simulink model "VisionVehicleDetectorTestBench"  (R2024b)
settings: Solver=FixedStepAuto  StartTime=0.0  StopTime=scenario.StopTime  RelTol=1e-3
PostLoadFcn:
  | helperSLVisionVehicleDetectorSetup
values from neighbouring files (symbols this model uses):
  vehSim3D = repmat(         struct(             'Length', 0,             'RearOverhang', 0,             'InitialPos',[0 0 0],             'InitialRot',[0 0 0]),         numVehicles,1)    [helperSLVisionVehicleDetectorSetup.m]
undefined symbols (not defined in the file or in its folder): Sim3dSensor, Ts
libraries: drivingscenarioandsensors x8, sim3dautolib x6, sim3dcameralib x1, sim3dlib x1
CloseFcn:
  | helperSLVisionVehicleDetectorCleanUp
settings Model: SILPILSystemUnderTest=refmodels  Creator=The MathWorks, Inc.  LastModifiedBy=The MathWorks, Inc.
settings SolverCC: AlgebraicLoopSolver=TrustRegion  MaxZcPerStep=1
settings DataIOCC: SaveFormat=StructureWithTime  SaveOutput=off  DSMLogging=off  SaveTime=off
settings OptimizationCC: DefaultParameterBehavior=Inlined  EnhancedBackFolding=on  PassReuseOutputArgsAs=Individual arguments  ZeroExternalMemoryAtStartup=off  ZeroInternalMemoryAtStartup=off  InitFltsAndDblsToZero=on  OptimizeBlockOrder=speed  DifferentSizesBufferReuse=on  OptimizationCustomize=off  EfficientTunableParamExpr=on
settings DebuggingCC: ParameterTunabilityLossMsg=error  UnconnectedInputMsg=warning  UnconnectedOutputMsg=warning  UnconnectedLineMsg=warning  SubsystemReferenceDiagnosticForUnitTest=warning
settings HardwareCC: ProdLongLongMode=on  TargetLongLongMode=on
settings ModelReferenceCC: EnableRefExpFcnMdlSchedulingChecks=on
settings SFSimCC: SimTargetLang=C++
settings RTWCC: Description=Embedded Coder  SystemTargetFile=ert.tlc  TemplateMakefile=ert_default_tmf  CodeExecutionProfiling=on  CodeProfilingSaveOptions=AllData  TargetLang=C++  GPUComputeCapability=3.5  DLArmComputeVersion=19.05
settings CodeAppCC: ForceParamTrailComments=on  IgnoreCustomStorageClasses=off  OperatorAnnotations=on  SimulinkDataObjDesc=on  SFDataObjDesc=on  InsertBlockDesc=on
settings ERTTargetCC: TargetLangStandard=C++03 (ISO)  GenerateSampleERTMain=on  CodeInterfacePackaging=C++ class  SupportVariableSizeSignals=on  RootIOFormat=Structure reference  ERTCustomFileTemplate=example_file_process.tlc  DynamicArrayContainerType=coder::array
settings ConfigComp: CovScope=ReferencedModels  CovIncludeTopModel=off  CovExternalEMLEnable=off  CovSFcnEnable=off

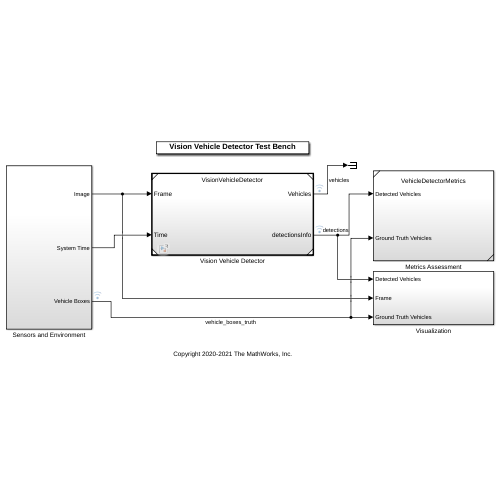
[thumbnail: Simulink's stored preview of the top-level diagram]
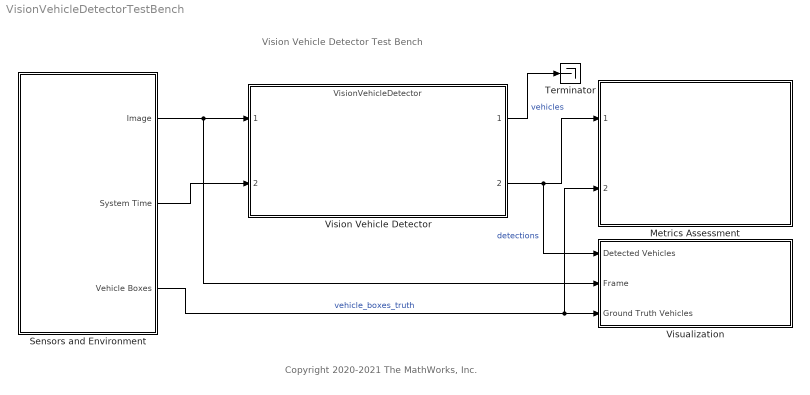
== system VisionVehicleDetectorTestBench ==
  note: Copyright 2020-2021 The MathWorks, Inc.
  note: Vision Vehicle Detector Test Bench
  Metrics Assessment : Subsystem  ReferencedSubsystem=VehicleDetectorMetrics
  Sensors and Environment : Subsystem
  Terminator : Terminator
  Vision Vehicle Detector : ModelReference  ModelNameDialog=VisionVehicleDetector.slx  SimulationMode=Normal  CodeInterface=Top model  ModelReferenceVersion=9.0
  Visualization : Subsystem
  wires:
  Sensors and Environment/3(Vehicle Boxes) -> Visualization/3(Ground Truth Vehicles), Metrics Assessment/2  "vehicle_boxes_truth"
  Sensors and Environment/1(Image) -> Vision Vehicle Detector/1, Visualization/2(Frame)
  Sensors and Environment/2(System Time) -> Vision Vehicle Detector/2
  Vision Vehicle Detector/1 -> Terminator/1  "vehicles"
  Vision Vehicle Detector/2 -> Metrics Assessment/1, Visualization/1(Detected Vehicles)  "detections"

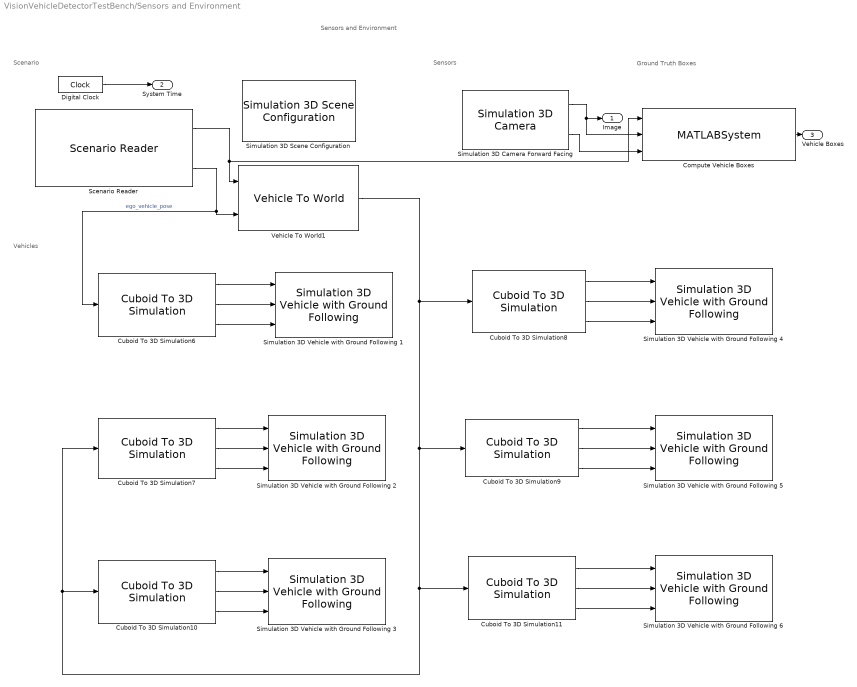
== system VisionVehicleDetectorTestBench/Sensors and Environment ==
  note: Sensors and Environment
  note: Ground Truth Boxes
  note: Sensors
  note: Vehicles
  note: Scenario
  Compute Vehicle Boxes : MATLABSystem  System=HelperComputeGroundTruthBoxes  VehicleDimensions=dimensions  Camera=camera  SimulateUsing=Interpreted execution
      mask Type: HelperComputeGroundTruthBoxes
      mask Display:
      | disp('HelperComputeGroundTruthBoxes');
      | port_label('input',1,'actorPositions');
      | port_label('input',2,'frame');
      | port_label('input',3,'labelledFrame');
      | port_label('output',1,'BBoxes');
  Cuboid To 3D Simulation10 : drivingscenarioandsensors/Cuboid To 3D Simulation  SpecifyActorID=on  ActorIDToConvert=3  SimulateUsing=Interpreted execution
  Cuboid To 3D Simulation11 : drivingscenarioandsensors/Cuboid To 3D Simulation  SpecifyActorID=on  ActorIDToConvert=6  SimulateUsing=Interpreted execution
  Cuboid To 3D Simulation6 : drivingscenarioandsensors/Cuboid To 3D Simulation  SpecifyActorID=off  ActorIDToConvert=1  SimulateUsing=Interpreted execution
  Cuboid To 3D Simulation7 : drivingscenarioandsensors/Cuboid To 3D Simulation  SpecifyActorID=on  ActorIDToConvert=2  SimulateUsing=Interpreted execution
  Cuboid To 3D Simulation8 : drivingscenarioandsensors/Cuboid To 3D Simulation  SpecifyActorID=on  ActorIDToConvert=4  SimulateUsing=Interpreted execution
  Cuboid To 3D Simulation9 : drivingscenarioandsensors/Cuboid To 3D Simulation  SpecifyActorID=on  ActorIDToConvert=5  SimulateUsing=Interpreted execution
  Digital Clock : DigitalClock  SampleTime=0.1
  Scenario Reader : drivingscenarioandsensors/Scenario Reader  ScenarioSource=From workspace  ScenarioFileName=dblLaneChangeDrivingScenario.mat  ScenarioVariableName=scenario  OutputCoordinateSystem=Vehicle coordinates  EgoVehicleSource=Scenario  EgoVehicleActorID=1  OrientVehiclesOnRoad=off  OutputEgoVehiclePose=on  OutputEgoVehicleState=off  SampleTime=0.1  LaneBoundaryOutput=None  LaneBoundaryDistance=0:0.5:70  LaneBoundaryLocation=Center of lane markings  BusNameSource=Auto  BusName=BusActors  BusNumActorsSource=Scenario  BusNumActors=100  BusName2Source=Auto  BusName2=BusLaneBoundaries  BusNumLaneBoundariesSource=Scenario  BusNumLaneBoundaries=10  BusName3Source=Auto  BusName3=BusEgoActor  BusName4Source=Auto  BusName4=BusEgoState  ShowCoordinateLabels=on  SimulateUsing=Interpreted execution
  Simulation 3D Camera Forward Facing : sim3dcameralib/Simulation 3D Camera  Priority=1  sensorTag=Sim3dSensor�  sensorId=1  sensorName=Sim3dSensor�  vehTagList={'Scene Origin';'SimulinkVehicle1';'SimulinkVehicle2';'SimulinkVehicle3';'SimulinkVehicle4';'SimulinkVehicle5';'SimulinkVehicle6'}  vehTag=SimulinkVehicle1  mountLoc=Origin  offsetFlag=on  tmountOffset=camera.PositionSim3d  extTmount=off  rmountOffset=camera.Rotation  extRmount=off  FocalLength=camera.FocalLength  OpticalCenter=camera.PrincipalPoint  ImageSize=camera.ImageSize  RadialDistortion=[0, 0]  TangentialDistortion=[0, 0]  SensorSkew=0  DepthOutportEnabled=off  SemanticOutportEnabled=on  TransformOutportEnabled=off  SampleTime=-1  mountPoint=[0.57 0 1.2]  mountOrientation=[0 0 0]  aMode=3  ID=1
      settings: LibrarySourceBlock=drivingsim3d/Simulation 3D Camera
      settings: AttributesFormatString=|
      | -------------------------------------
      | ImageSize = %<ImageSize>
      | OpticalCenter = %<OpticalCenter>
      | FocalLength = %<FocalLength>
      | RadialDistortion = %<RadialDistortion>
      | mountLoc = %<mountLoc>
      | tmountOffset = %<tmountOffset>
      | rmountOffset = %<rmountOffset>
  Simulation 3D Scene Configuration : sim3dlib/Simulation 3D Scene Configuration  Priority=0  ProjectFormat=Default Scenes  SceneDesc=Curved road  ProjectName=/mathworks/devel/bat/filer/batfs2566-0/Bdoc24b.2855429/build/runnable/matlab/toolbox/shared/sim3d_projects/automotive_project_linux/UE/LinuxNoEditor/VehicleSimulation.sh  ScenePath=/Game/Maps/HwStrght  EnableOpenDRIVE=off  vehTagList={'Scene Origin';'SimulinkVehicle1';'SimulinkVehicle2';'SimulinkVehicle3';'SimulinkVehicle4';'SimulinkVehicle5';'SimulinkVehicle6'}  vehTag=SimulinkVehicle1  FreeCameraInitialTranslation=[0, 0, 0]  FreeCameraDefaultInitialTranslation=[-6, 0, 2]  FreeCameraInitialRotation=[0, 0, 0]  FreeCameraDefaultInitialRotation=[0, -15, 0]  OpVisEn=off  Ts=0.1  EnableWindow=on  EnableRemoteAccess=off  EnableWeather=off  SunAzimuth=90  SunAltitude=40.0  EnableGeospatialSun=off  Latitude=0  Longitude=0  Date=2023-01-01  Time=10:30:00  GeoTimeZone=-5.0  SunDaylightSaving=off  wind=1  clouds=10  EnableVolumetricClouds=off  CloudCoverage=0  CloudAltitude=6  fog=0  rain=0  RaindropsEffect=off  SnowDensity=0  EnableGeospatial=off  UseTrueOrigin=off  OriginHeight=200  OriginLatitude=40.744652  OriginLongitude=-73.988864  MapStyle=Aerial  AdditionalAssetIDs=[]  UseAdvancedSunSky=off  SolarTime=11  TimeZone=-5  Day=21  Month=9  Year=2022  UseDaylightSavingTime=on  DSTStartDay=10  DSTStartMonth=3  DSTEndDay=3  DSTEndMonth=11  DSTSwitchHour=2  sensorTag=MainCamera2  sensorId=2  sensorName=MainCamera2  mountLoc=Origin  offsetFlag=off  tmountOffset=[0, 0, 0]  rmountOffset=[0, 0, 0]  HorizontalResolution=1280  VerticalResolution=720  HorizontalFOV=60  mountPoint=[0 0 0]  mountOrientation=[0 0 0]  aMode=3  ID=2  GeoTrigger=Inactive
      settings: AttributesFormatString=SceneName = %<SceneDesc>  LibrarySourceBlock=drivingsim3d/Simulation 3D Scene Configuration
  Simulation 3D Vehicle with Ground Following 1 : sim3dautolib/Simulation 3D Vehicle with Ground Following  Priority=-1  PassVehMesh=Sedan  MeshPath=/MathWorksSimulation/Vehicles/Muscle/Meshes/SK_MuscleCar.SK_MuscleCar  TrackWidth=1.9  WheelBase=3  WheelRadius=0.35  VehColor=Blue  InitialPos=vehSim3D(1).InitialPos  InitialRot=vehSim3D(1).InitialRot  ActorName=SimulinkVehicle1  SampleTime=-1  ActorType=SimulinkVehicle  ID=1  aMode=3  ActorTag=SimulinkVehicle1  CoordinateScheme=ISO  VehLightsControl=off  HeadlightColor=[ 1, 1, 1 ]  HighBeamIntensity=100000  LowBeamIntensity=60000  HighBeamConeAngle=70  LowBeamConeAngle=70  LeftHeadlightOrientation=[ 0, 0 ]  RightHeadlightOrientation=[ 0, 0 ]  BrakelightIntensity=500  ReverselightIntensity=500  SignallightIntensity=500  SignallightPeriod=1  SignalPulseWidth=50  TransformOutportEnabled=off
      settings: LibrarySourceBlock=drivingsim3d/Simulation 3D Vehicle with Ground Following
      settings: AttributesFormatString=|
      | --------------------------------------
      | ActorName = %<ActorName>
      | PassVehMesh = %<PassVehMesh>
      | VehColor = %<VehColor>
  Simulation 3D Vehicle with Ground Following 2 : sim3dautolib/Simulation 3D Vehicle with Ground Following  Priority=-1  PassVehMesh=Sedan  MeshPath=/MathWorksSimulation/Vehicles/Muscle/Meshes/SK_MuscleCar.SK_MuscleCar  TrackWidth=1.9  WheelBase=3  WheelRadius=0.35  VehColor=Red  InitialPos=vehSim3D(2).InitialPos  InitialRot=vehSim3D(2).InitialRot  ActorName=SimulinkVehicle2  SampleTime=-1  ActorType=SimulinkVehicle  ID=2  aMode=3  ActorTag=SimulinkVehicle2  CoordinateScheme=ISO  VehLightsControl=off  HeadlightColor=[ 1, 1, 1 ]  HighBeamIntensity=100000  LowBeamIntensity=60000  HighBeamConeAngle=70  LowBeamConeAngle=70  LeftHeadlightOrientation=[ 0, 0 ]  RightHeadlightOrientation=[ 0, 0 ]  BrakelightIntensity=500  ReverselightIntensity=500  SignallightIntensity=500  SignallightPeriod=1  SignalPulseWidth=50  TransformOutportEnabled=off
      settings: LibrarySourceBlock=drivingsim3d/Simulation 3D Vehicle with Ground Following
      settings: AttributesFormatString=|
      | --------------------------------------
      | ActorName = %<ActorName>
      | PassVehMesh = %<PassVehMesh>
      | VehColor = %<VehColor>
  Simulation 3D Vehicle with Ground Following 3 : sim3dautolib/Simulation 3D Vehicle with Ground Following  Priority=-1  PassVehMesh=Muscle car  MeshPath=/MathWorksSimulation/Vehicles/Muscle/Meshes/SK_MuscleCar.SK_MuscleCar  TrackWidth=1.9  WheelBase=3  WheelRadius=0.35  VehColor=Black  InitialPos=vehSim3D(3).InitialPos  InitialRot=vehSim3D(3).InitialRot  ActorName=SimulinkVehicle3  SampleTime=-1  ActorType=SimulinkVehicle  ID=3  aMode=3  ActorTag=SimulinkVehicle3  CoordinateScheme=ISO  VehLightsControl=off  HeadlightColor=[ 1, 1, 1 ]  HighBeamIntensity=100000  LowBeamIntensity=60000  HighBeamConeAngle=70  LowBeamConeAngle=70  LeftHeadlightOrientation=[ 0, 0 ]  RightHeadlightOrientation=[ 0, 0 ]  BrakelightIntensity=500  ReverselightIntensity=500  SignallightIntensity=500  SignallightPeriod=1  SignalPulseWidth=50  TransformOutportEnabled=off
      settings: LibrarySourceBlock=drivingsim3d/Simulation 3D Vehicle with Ground Following
      settings: AttributesFormatString=|
      | --------------------------------------
      | ActorName = %<ActorName>
      | PassVehMesh = %<PassVehMesh>
      | VehColor = %<VehColor>
  "Simulation 3D Vehicle with Ground Following 4 " : sim3dautolib/Simulation 3D Vehicle with Ground Following  Priority=-1  PassVehMesh=Muscle car  MeshPath=/MathWorksSimulation/Vehicles/Muscle/Meshes/SK_MuscleCar.SK_MuscleCar  TrackWidth=1.9  WheelBase=3  WheelRadius=0.35  VehColor=Black  InitialPos=vehSim3D(4).InitialPos  InitialRot=vehSim3D(4).InitialRot  ActorName=SimulinkVehicle4  SampleTime=-1  ActorType=SimulinkVehicle  ID=4  aMode=3  ActorTag=SimulinkVehicle4  CoordinateScheme=ISO  VehLightsControl=off  HeadlightColor=[ 1, 1, 1 ]  HighBeamIntensity=100000  LowBeamIntensity=60000  HighBeamConeAngle=70  LowBeamConeAngle=70  LeftHeadlightOrientation=[ 0, 0 ]  RightHeadlightOrientation=[ 0, 0 ]  BrakelightIntensity=500  ReverselightIntensity=500  SignallightIntensity=500  SignallightPeriod=1  SignalPulseWidth=50  TransformOutportEnabled=off
      settings: LibrarySourceBlock=drivingsim3d/Simulation 3D Vehicle with Ground Following
      settings: AttributesFormatString=|
      | --------------------------------------
      | ActorName = %<ActorName>
      | PassVehMesh = %<PassVehMesh>
      | VehColor = %<VehColor>
  Simulation 3D Vehicle with Ground Following 5 : sim3dautolib/Simulation 3D Vehicle with Ground Following  Priority=-1  PassVehMesh=Small pickup truck  MeshPath=/MathWorksSimulation/Vehicles/Muscle/Meshes/SK_MuscleCar.SK_MuscleCar  TrackWidth=1.9  WheelBase=3  WheelRadius=0.35  VehColor=Green  InitialPos=vehSim3D(5).InitialPos  InitialRot=vehSim3D(5).InitialRot  ActorName=SimulinkVehicle5  SampleTime=-1  ActorType=SimulinkVehicle  ID=5  aMode=3  ActorTag=SimulinkVehicle5  CoordinateScheme=ISO  VehLightsControl=off  HeadlightColor=[ 1, 1, 1 ]  HighBeamIntensity=100000  LowBeamIntensity=60000  HighBeamConeAngle=70  LowBeamConeAngle=70  LeftHeadlightOrientation=[ 0, 0 ]  RightHeadlightOrientation=[ 0, 0 ]  BrakelightIntensity=500  ReverselightIntensity=500  SignallightIntensity=500  SignallightPeriod=1  SignalPulseWidth=50  TransformOutportEnabled=off
      settings: LibrarySourceBlock=drivingsim3d/Simulation 3D Vehicle with Ground Following
      settings: AttributesFormatString=|
      | --------------------------------------
      | ActorName = %<ActorName>
      | PassVehMesh = %<PassVehMesh>
      | VehColor = %<VehColor>
  Simulation 3D Vehicle with Ground Following 6 : sim3dautolib/Simulation 3D Vehicle with Ground Following  Priority=-1  PassVehMesh=Sport utility vehicle  MeshPath=/MathWorksSimulation/Vehicles/Muscle/Meshes/SK_MuscleCar.SK_MuscleCar  TrackWidth=1.9  WheelBase=3  WheelRadius=0.35  VehColor=Blue  InitialPos=vehSim3D(6).InitialPos  InitialRot=vehSim3D(6).InitialRot  ActorName=SimulinkVehicle6  SampleTime=-1  ActorType=SimulinkVehicle  ID=6  aMode=3  ActorTag=SimulinkVehicle6  CoordinateScheme=ISO  VehLightsControl=off  HeadlightColor=[ 1, 1, 1 ]  HighBeamIntensity=100000  LowBeamIntensity=60000  HighBeamConeAngle=70  LowBeamConeAngle=70  LeftHeadlightOrientation=[ 0, 0 ]  RightHeadlightOrientation=[ 0, 0 ]  BrakelightIntensity=500  ReverselightIntensity=500  SignallightIntensity=500  SignallightPeriod=1  SignalPulseWidth=50  TransformOutportEnabled=off
      settings: LibrarySourceBlock=drivingsim3d/Simulation 3D Vehicle with Ground Following
      settings: AttributesFormatString=|
      | --------------------------------------
      | ActorName = %<ActorName>
      | PassVehMesh = %<PassVehMesh>
      | VehColor = %<VehColor>
  Vehicle To World1 : drivingscenarioandsensors/Vehicle To World  BusNameSource=Auto  BusName=BusVehicleToWorldActors  SimulateUsing=Interpreted execution
  Image : Outport  SampleTime=Ts  VectorParamsAs1DForOutWhenUnconnected=off
  System Time : Outport  Port=2
  Vehicle Boxes : Outport  Port=3
  wires:
  Simulation 3D Camera Forward Facing/1 -> Compute Vehicle Boxes/2, Image/1
  Cuboid To 3D Simulation7/2 -> Simulation 3D Vehicle with Ground Following 2/2
  Vehicle To World1/1 -> Cuboid To 3D Simulation8/1, Cuboid To 3D Simulation9/1, Cuboid To 3D Simulation11/1, Cuboid To 3D Simulation7/1, Cuboid To 3D Simulation10/1
  Cuboid To 3D Simulation7/3 -> Simulation 3D Vehicle with Ground Following 2/3
  Cuboid To 3D Simulation11/1 -> Simulation 3D Vehicle with Ground Following 6/1
  Scenario Reader/1 -> Compute Vehicle Boxes/1, Vehicle To World1/1
  Cuboid To 3D Simulation9/1 -> Simulation 3D Vehicle with Ground Following 5/1
  Cuboid To 3D Simulation9/2 -> Simulation 3D Vehicle with Ground Following 5/2
  Cuboid To 3D Simulation11/3 -> Simulation 3D Vehicle with Ground Following 6/3
  Cuboid To 3D Simulation10/3 -> Simulation 3D Vehicle with Ground Following 3/3
  Cuboid To 3D Simulation6/2 -> Simulation 3D Vehicle with Ground Following 1/2
  Cuboid To 3D Simulation11/2 -> Simulation 3D Vehicle with Ground Following 6/2
  Cuboid To 3D Simulation10/2 -> Simulation 3D Vehicle with Ground Following 3/2
  Cuboid To 3D Simulation10/1 -> Simulation 3D Vehicle with Ground Following 3/1
  Cuboid To 3D Simulation8/1 -> "Simulation 3D Vehicle with Ground Following 4 "/1
  Cuboid To 3D Simulation6/3 -> Simulation 3D Vehicle with Ground Following 1/3
  Cuboid To 3D Simulation9/3 -> Simulation 3D Vehicle with Ground Following 5/3
  Cuboid To 3D Simulation8/2 -> "Simulation 3D Vehicle with Ground Following 4 "/2
  Cuboid To 3D Simulation8/3 -> "Simulation 3D Vehicle with Ground Following 4 "/3
  Cuboid To 3D Simulation6/1 -> Simulation 3D Vehicle with Ground Following 1/1
  Cuboid To 3D Simulation7/1 -> Simulation 3D Vehicle with Ground Following 2/1
  Compute Vehicle Boxes/1 -> Vehicle Boxes/1
  Digital Clock/1 -> System Time/1
  Simulation 3D Camera Forward Facing/2 -> Compute Vehicle Boxes/3
  Scenario Reader/2 -> Vehicle To World1/2, Cuboid To 3D Simulation6/1  "ego_vehicle_pose"

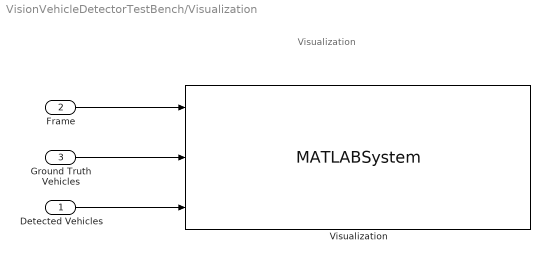
== system VisionVehicleDetectorTestBench/Visualization ==
  note: Visualization
  Detected Vehicles : Inport
  Frame : Inport  Port=2
  Ground Truth Vehicles : Inport  Port=3
  Visualization : MATLABSystem  System=HelperVisualizeVehicles  EnableTruthDisplay=off  Camera=camera
      mask Type: HelperVisualizeVehicles
      mask Display:
      | disp('HelperVisualizeVehicles');
      | port_label('input',1,'frame');
      | port_label('input',2,'groundTruthVehicles');
      | port_label('input',3,'detectedVehicles');
  wires:
  Frame/1 -> Visualization/1
  Ground Truth Vehicles/1 -> Visualization/2
  Detected Vehicles/1 -> Visualization/3
